simulink model "test_net"  (R2024b)
settings: Solver=VariableStepAuto  StartTime=0.0  StopTime=10.0  RelTol=1e-3
settings Model: Creator=xpess  LastModifiedBy=xpess

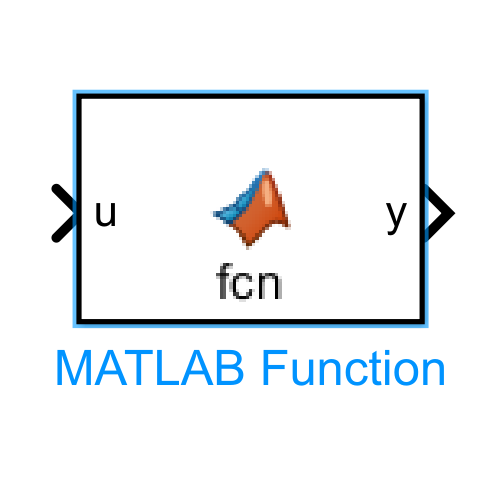
[thumbnail: Simulink's stored preview of the top-level diagram]
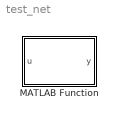
== system test_net ==
  MATLAB Function : MATLAB Function  TreatAsAtomicUnit=on

== matlab function test_net/MATLAB Function ==
  data: u input; y output
function y = fcn(u)
    predict(net,u)
y = predict(net,u);
